simulink model "nonlinear_inverted_pendulum_simulation_indirect"  (R2016b)
settings: Solver=ode15s  StartTime=0.0  StopTime=10.0  RelTol=1e-3  EnableMultiTasking=on
values from neighbouring files (symbols this model uses):
  A = sys.A    [LoopGain.m]    (also in dcontrold_dir.m = sys_d.A; main.m = [                   0,                                      ; simulation.m)
  B = sys.B    [LoopGain.m]    (also in dcontrold_dir.m = sys_d.B; main.m = [                   0; ( 3*Km*Vs)/(LinkMass*(LinkLength^2)*R; simulation.m)
  b_motor = 0    [main.m]
  C = sys.C    [LoopGain.m]    (also in dcontrold_dir.m = sys_d.C; main.m = [                   1,                                      ; simulation.m)
  Ctrl_FB = minreal( -tf( ss(A - L*C - B*K, L, K, zeros(nInputs,nOutputs))))    [simulation.m]
  g = 9.81    [main.m]
  J_total = 3.97396e-05    [InvPendModel.mat]    (also in main.m = 8.7667803511e-05)
  K = place(A,B,Kp)    [dcontrold_dir.m]    (also in dcontrold_ind.m = place(A, B, desFbPoles); sysStateEstimatorFeedbackWithModel.m = Kaug(1:nStates))
  Kb = Km    (= 0.0265805280355)    [main.m]
  Km = Vs/kappa_id    (= 0.0265805280355)    [main.m]    (also in sysStateEstimatorFeedbackWithModel.m = Kaug(nStates + 1:end))
  L = place(A',C',Lp)'    [dcontrold_dir.m]    (also in dcontrold_ind.m = place(A', C', desObsPoles).')
  L_motor = 0.24E-3    (= 0.00024)    [main.m]
  LinkLength = 0.0508    [InvPendModel.mat]    (also in main.m = 0.07539)
  LinkMass = 0.045    [InvPendModel.mat]    (also in main.m = 0.04573)
  N = 1 / (Cc * inv(eye(nStates)-sysCL.A) * Bc)    [analysis.m]
  R_motor = tau_id*Km^2 / J_total    (= 1.619075196)    [main.m]
  Ts = sys.Ts    [LoopGain.m]    (also in analysis.m = 1/Hz; main.m = T(end); simulation.m = 0.001; system_id_batch.m = 0.001)
  Vs = 12    [main.m]
libraries: cstblocks x2
settings Model: Creator=Martin  LastModifiedBy=preston
settings OptimizationCC: LifeSpan=inf
settings DebuggingCC: SFUnexpectedBacktrackingDiag=warning  SFNoUnconditionalDefaultTransitionDiag=warning  SFExecutionAtInitializationDiag=none
settings GRTTargetCC: TargetLangStandard=C89/C90 (ANSI)  GeneratePreprocessorConditionals=Disable all
settings ConfigComp: CovMetricSettings=dw  CovHtmlReporting=on  CovSaveCumulativeToWorkspaceVar=on  CovSaveSingleToWorkspaceVar=on  CovExternalEMLEnable=off

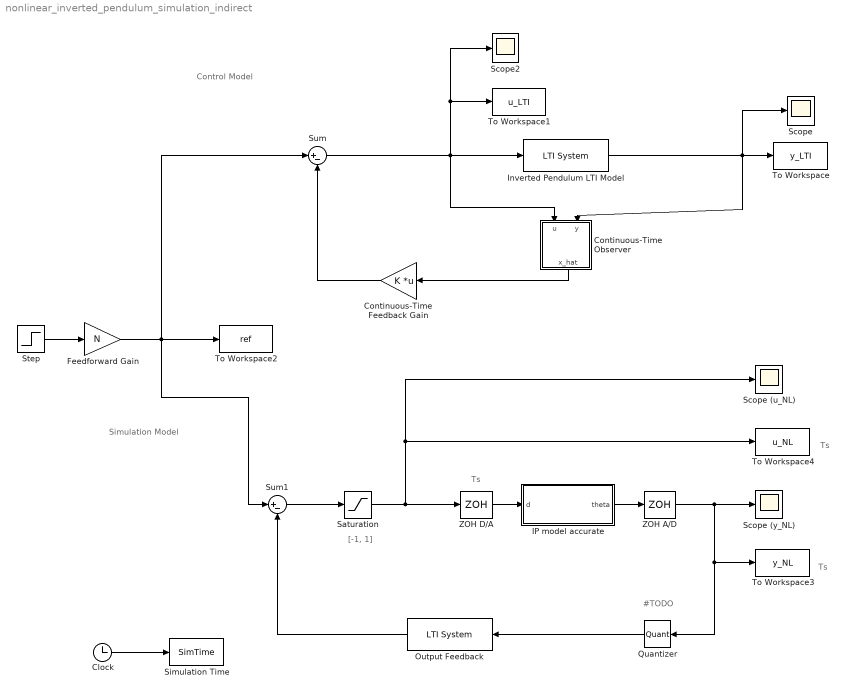
== system nonlinear_inverted_pendulum_simulation_indirect ==
  note: Control Model
  note: Simulation Model
  note: Ts
  note: Ts
  note: #TODO
  note: [-1, 1]
  note: Ts
  Clock : Clock
  Continuous-Time Feedback Gain : Gain  Gain=K  Multiplication=Matrix(K*u)
  Continuous-Time Observer : Subsystem
  Feedforward Gain : Gain  Gain=N
  IP model accurate : Subsystem
  Inverted Pendulum LTI Model : cstblocks/LTI System  sys=sysP  IC=[]
  Output Feedback : cstblocks/LTI System  sys=-Ctrl_FB  IC=[]
  Quantizer : Quantizer  QuantizationInterval=QzrLvl
  Saturation : Saturate  UpperLimit=1  LowerLimit=-1
  Scope : Scope
  Scope (u_NL) : Scope
  Scope (y_NL) : Scope
  Scope2 : Scope
  Simulation Time : ToWorkspace  VariableName=SimTime  SampleTime=-1
  Step : Step  After=.2  SampleTime=0
  Sum : Sum  Inputs=|+-
  Sum1 : Sum  Inputs=|+-
  To Workspace : ToWorkspace  VariableName=y_LTI  SaveFormat=Timeseries  SampleTime=Ts
  To Workspace1 : ToWorkspace  VariableName=u_LTI  SaveFormat=Timeseries  SampleTime=Ts
  To Workspace2 : ToWorkspace  VariableName=ref  SaveFormat=Timeseries  SampleTime=Ts
  To Workspace3 : ToWorkspace  VariableName=y_NL  SaveFormat=Timeseries  SampleTime=Ts
  To Workspace4 : ToWorkspace  VariableName=u_NL  SaveFormat=Timeseries  SampleTime=Ts
  ZOH A/D : ZeroOrderHold  SampleTime=Ts
  ZOH D/A : ZeroOrderHold  SampleTime=Ts
  wires:
  Feedforward Gain/1 -> Sum1/1, To Workspace2/1, Sum/1
  Inverted Pendulum LTI Model/1 -> Continuous-Time Observer/2(y), To Workspace/1, Scope/1
  Clock/1 -> Simulation Time/1
  Sum/1 -> Inverted Pendulum LTI Model/1, Continuous-Time Observer/1(u), Scope2/1, To Workspace1/1
  Continuous-Time Feedback Gain/1 -> Sum/2
  Continuous-Time Observer/1(x_hat) -> Continuous-Time Feedback Gain/1
  Step/1 -> Feedforward Gain/1
  ZOH D/A/1 -> IP model accurate/1(d)
  IP model accurate/1(theta) -> ZOH A/D/1
  Saturation/1 -> To Workspace4/1, Scope (u_NL)/1, ZOH D/A/1
  Sum1/1 -> Saturation/1
  ZOH A/D/1 -> Quantizer/1, To Workspace3/1, Scope (y_NL)/1
  Quantizer/1 -> Output Feedback/1
  Output Feedback/1 -> Sum1/2

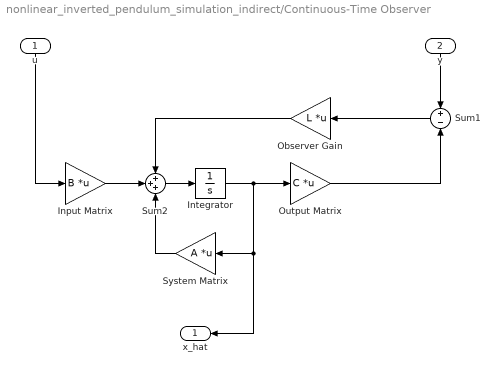
== system nonlinear_inverted_pendulum_simulation_indirect/Continuous-Time Observer ==
  u : Inport
  y : Inport  Port=2
  Input Matrix : Gain  Gain=B  Multiplication=Matrix(K*u)
  Integrator : Integrator
  Observer Gain : Gain  Gain=L  Multiplication=Matrix(K*u)
  Output Matrix : Gain  Gain=C  Multiplication=Matrix(K*u)
  Sum1 : Sum  Inputs=+|-
  Sum2 : Sum  Inputs=+++
  System Matrix : Gain  Gain=A  Multiplication=Matrix(K*u)
  x_hat : Outport
  wires:
  y/1 -> Sum1/1
  Integrator/1 -> Output Matrix/1, System Matrix/1, x_hat/1
  u/1 -> Input Matrix/1
  Observer Gain/1 -> Sum2/1
  Input Matrix/1 -> Sum2/2
  Output Matrix/1 -> Sum1/2
  Sum2/1 -> Integrator/1
  System Matrix/1 -> Sum2/3
  Sum1/1 -> Observer Gain/1

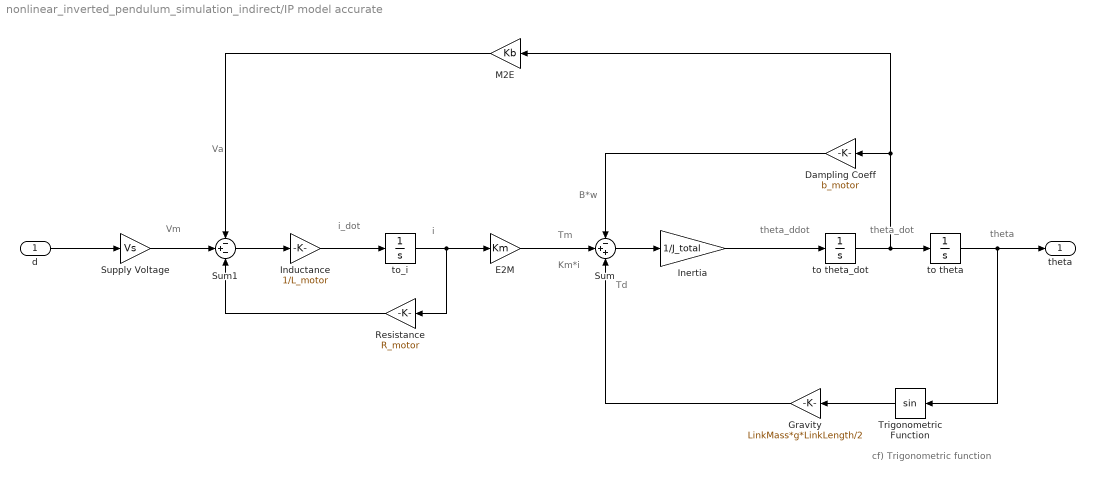
== system nonlinear_inverted_pendulum_simulation_indirect/IP model accurate ==
  note: Va
  note: Vm
  note: i_dot
  note: B*w
  note: Td
  note: Km*i
  note: Tm
  note: i
  note: cf) Trigonometric
      | function
  note: theta_ddot
  note: theta
  note: theta_dot
  d : Inport
  Dampling Coeff : Gain  Gain=b_motor
  E2M : Gain  Gain=Km
  Gravity : Gain  Gain=LinkMass*g*LinkLength/2
  Inductance : Gain  Gain=1/L_motor
  Inertia : Gain  Gain=1/J_total
  M2E : Gain  Gain=Kb
  Resistance : Gain  Gain=R_motor
  Sum : Sum  Inputs=-++
  Sum1 : Sum  Inputs=-+-
  Supply Voltage : Gain  Gain=Vs
  Trigonometric Function : Trigonometry
  to theta : Integrator
  to theta_dot : Integrator
  to_i : Integrator
  theta : Outport
  wires:
  to theta_dot/1 -> to theta/1, M2E/1, Dampling Coeff/1
  to theta/1 -> Trigonometric Function/1, theta/1
  Trigonometric Function/1 -> Gravity/1
  E2M/1 -> Sum/2
  Dampling Coeff/1 -> Sum/1
  Gravity/1 -> Sum/3
  to_i/1 -> Resistance/1, E2M/1
  Resistance/1 -> Sum1/3
  d/1 -> Supply Voltage/1
  Supply Voltage/1 -> Sum1/2
  M2E/1 -> Sum1/1
  Sum1/1 -> Inductance/1
  Inductance/1 -> to_i/1
  Sum/1 -> Inertia/1
  Inertia/1 -> to theta_dot/1
